simulink model "module_12s"  (R2024b)
settings: Solver=ode4  StartTime=0.0  StopTime=T_stop  FixedStep=0.1  RelTol=1e-3
settings Model: Creator=rayen  LastModifiedBy=rayen
settings DebuggingCC: AlgebraicLoopMsg=error

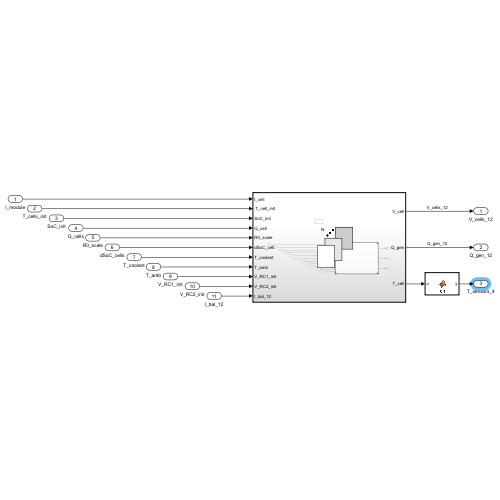
[thumbnail: Simulink's stored preview of the top-level diagram]
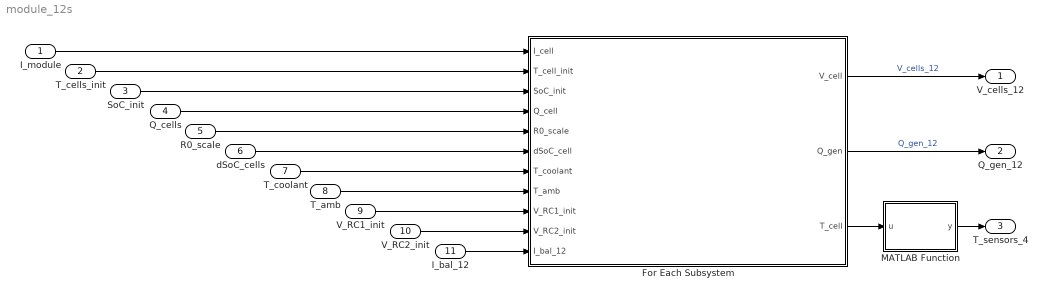
== system module_12s ==
  I_module : Inport  OutDataTypeStr=double
  T_cells_init : Inport  Port=2  OutDataTypeStr=double
  SoC_init : Inport  Port=3  OutDataTypeStr=double
  Q_cells : Inport  Port=4  OutDataTypeStr=double
  R0_scale : Inport  Port=5  OutDataTypeStr=double
  dSoC_cells : Inport  Port=6  OutDataTypeStr=double
  T_coolant : Inport  Port=7  OutDataTypeStr=double
  T_amb : Inport  Port=8  OutDataTypeStr=double
  V_RC1_init : Inport  Port=9  OutDataTypeStr=double
  V_RC2_init : Inport  Port=10  OutDataTypeStr=double
  I_bal_12 : Inport  Port=11  OutDataTypeStr=double
  For Each Subsystem : Subsystem  TreatAsAtomicUnit=on
  MATLAB Function : MATLAB Function  TreatAsAtomicUnit=on
  V_cells_12 : Outport  OutDataTypeStr=double  PortDimensions=12
  Q_gen_12 : Outport  Port=2  OutDataTypeStr=double  PortDimensions=12
  T_sensors_4 : Outport  Port=3  OutDataTypeStr=double
  wires:
  dSoC_cells/1 -> For Each Subsystem/6(dSoC_cell)
  R0_scale/1 -> For Each Subsystem/5(R0_scale)
  Q_cells/1 -> For Each Subsystem/4(Q_cell)
  SoC_init/1 -> For Each Subsystem/3(SoC_init)
  T_cells_init/1 -> For Each Subsystem/2(" T_cell_init")
  I_module/1 -> For Each Subsystem/1(I_cell)
  For Each Subsystem/1(V_cell) -> V_cells_12/1  "V_cells_12"
  T_coolant/1 -> For Each Subsystem/7(T_coolant)
  T_amb/1 -> For Each Subsystem/8(T_amb)
  V_RC1_init/1 -> For Each Subsystem/9(V_RC1_init)
  V_RC2_init/1 -> For Each Subsystem/10(V_RC2_init)
  I_bal_12/1 -> For Each Subsystem/11(I_bal_12)
  For Each Subsystem/3(T_cell) -> MATLAB Function/1(u)
  MATLAB Function/1(y) -> T_sensors_4/1
  For Each Subsystem/2(Q_gen) -> Q_gen_12/1  "Q_gen_12"

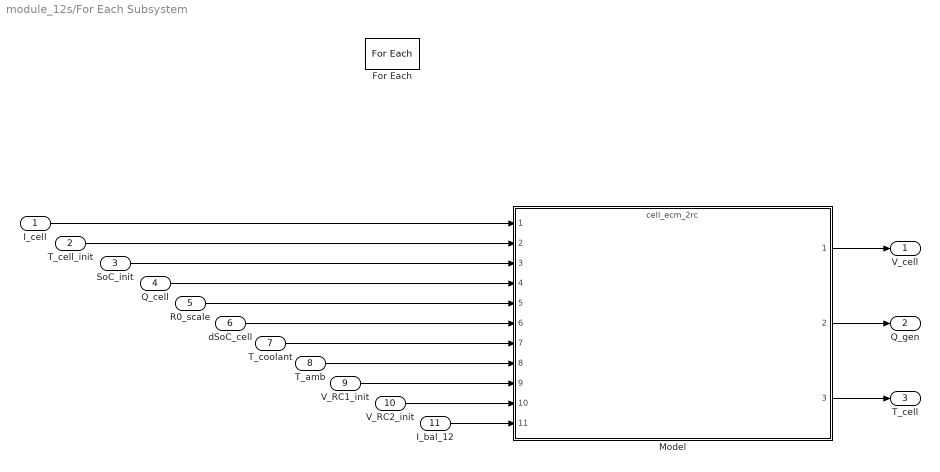
== system module_12s/For Each Subsystem ==
  I_cell : Inport
  " T_cell_init" : Inport  Port=2  Partition=on  PartitionDimension=1  PartitionWidth=1  PartitionOffset=0
  SoC_init : Inport  Port=3
  Q_cell : Inport  Port=4  Partition=on  PartitionDimension=1  PartitionWidth=1  PartitionOffset=0
  R0_scale : Inport  Port=5  Partition=on  PartitionDimension=1  PartitionWidth=1  PartitionOffset=0
  dSoC_cell : Inport  Port=6  Partition=on  PartitionDimension=1  PartitionWidth=1  PartitionOffset=0
  T_coolant : Inport  Port=7
  T_amb : Inport  Port=8
  V_RC1_init : Inport  Port=9
  V_RC2_init : Inport  Port=10
  I_bal_12 : Inport  Port=11  Partition=on  PartitionDimension=1  PartitionWidth=1  PartitionOffset=0
  For Each : ForEach  DisableCoverage=on
  Model : ModelReference  ModelNameDialog=cell_ecm_2rc.slx  ModelReferenceVersion=1.66
  V_cell : Outport  ConcatenationDimension=1
  Q_gen : Outport  Port=2  ConcatenationDimension=1
  T_cell : Outport  Port=3  ConcatenationDimension=1
  wires:
  Model/3 -> T_cell/1
  Model/1 -> V_cell/1
  I_cell/1 -> Model/1
  " T_cell_init"/1 -> Model/2
  SoC_init/1 -> Model/3
  Q_cell/1 -> Model/4
  R0_scale/1 -> Model/5
  dSoC_cell/1 -> Model/6
  T_coolant/1 -> Model/7
  T_amb/1 -> Model/8
  V_RC1_init/1 -> Model/9
  V_RC2_init/1 -> Model/10
  I_bal_12/1 -> Model/11
  Model/2 -> Q_gen/1

== matlab function module_12s/MATLAB Function ==
  data: u input; y output
function y = fcn(u)

y = zeros(4, 1);

for i = 1:4
    idx_start = (i - 1) * 3 + 1;    % 1, 4, 7, 10
    idx_end   = i * 3;              % 3, 6, 9, 12
    y(i) = mean(u(idx_start:idx_end));
end
